simulink model "ctrl_DP"  (R2016b)
settings: Solver=ode3  StartTime=0.0  StopTime=inf  FixedStep=0.01  RelTol=1e-3  EnableMultiTasking=on
values from neighbouring files (symbols this model uses):
  C = [C1;C2;C3;C4;C5;C6]    [initfile.m]
  D = 3.0/100    (= 0.03)    [initfile.m]
  eps_c = 5    [initfile.m]
  epsilon = 0.5    [initfile.m]
  hd = c2d(H1,0.01,'foh')    [initfile.m]
  hd2 = c2d(H2,0.01,'zoh')    [initfile.m]
  I_s = 25000 /747225    (= 0.0334571246947)    [initfile.m]
  k_cc = 1    [initfile.m]
  K_omega = 0.3    [initfile.m]
  K_q1f = 0.0113    [initfile.m]
  K_q1r = K_q1f    (= 0.0113)    [initfile.m]
  K_q2f = 0.0117    [initfile.m]
  K_q2r = K_q2f    (= 0.0117)    [initfile.m]
  K_q3f = 0.0113    [initfile.m]
  K_q3r = K_q3f    (= 0.0113)    [initfile.m]
  K_q4f = 0.0169    [initfile.m]
  K_q4r = K_q4f    (= 0.0169)    [initfile.m]
  K_q5f = 0.0144    [initfile.m]
  K_q5r = K_q5f    (= 0.0144)    [initfile.m]
  K_q6f = 0.0168    [initfile.m]
  K_q6r = K_q6f    (= 0.0168)    [initfile.m]
  K_T1f = 0.3763    [initfile.m]
  K_T1r = K_T1f    (= 0.3763)    [initfile.m]
  K_T2f = 0.3901    [initfile.m]
  K_T2r = K_T2f    (= 0.3901)    [initfile.m]
  K_T3f = 0.3776    [initfile.m]
  K_T3r = K_T3f    (= 0.3776)    [initfile.m]
  K_T4f = 0.5641    [initfile.m]
  K_T4r = K_T4f    (= 0.5641)    [initfile.m]
  K_T5f = 0.4799    [initfile.m]
  K_T5r = K_T5f    (= 0.4799)    [initfile.m]
  K_T6f = 0.5588    [initfile.m]
  K_T6r = K_T6f    (= 0.5588)    [initfile.m]
  Kp = 3.3    [initfile.m]
  Max_Acceleration = 5    [initfile.m]
  Max_rotation = 12*sqrt(lambda)    [initfile.m]
  Max_thrust = 1.5    [initfile.m]
  Min_thrust = -0.8    [initfile.m]
  n_c = 5    [initfile.m]
  n_max = 152    [initfile.m]
  p_cc = 0.5    [initfile.m]
  pwm_thr1_backward = coeffvalues(ForceToPWM)    [initfile.m]
  pwm_thr1_forward = coeffvalues(ForceToPWM)    [initfile.m]
  pwm_thr2_backward = coeffvalues(ForceToPWM)    [initfile.m]
  pwm_thr2_forward = coeffvalues(ForceToPWM)    [initfile.m]
  pwm_thr3_backward = coeffvalues(ForceToPWM)    [initfile.m]
  pwm_thr3_forward = coeffvalues(ForceToPWM)    [initfile.m]
  pwm_thr4_backward = coeffvalues(ForceToPWM)    [initfile.m]
  pwm_thr4_forward = coeffvalues(ForceToPWM)    [initfile.m]
  pwm_thr5_backward = coeffvalues(ForceToPWM)    [initfile.m]
  pwm_thr5_forward = coeffvalues(ForceToPWM)    [initfile.m]
  pwm_thr6_backward = coeffvalues(ForceToPWM)    [initfile.m]
  pwm_thr6_forward = coeffvalues(ForceToPWM)    [initfile.m]
  Q_f0 = 0.3    [initfile.m]
  r_cc = 4    [initfile.m]
  Rho = Rho_m    (= 1000)    [initfile.m]
  T_pinv = T'*inv(T*T')    [initfile.m]
undefined symbols (not defined in the file or in its folder): DiscIntNeverNeededParam, Q_max, Thruster
libraries: marine_gnc x8, simulink x6, simulink_extras x3
(part 2 of 6)

== system ctrl_DP/Output ==
  u : Inport
  alpha : Inport  Port=2
  Demux : Demux  Outputs=6
  Demux1 : Demux  Outputs=6
  alpha1 : S-Function  Priority=1  FunctionName=NIVeriStandIO  Parameters=width dtype portnum stime stype btype  SFunctionDeploymentMode=off  EnableBusSupport=off  mask(NI VeriStand Outport){portnum=1, width=-1, stime=-1, dtype=auto, stype=auto, btype=0}
      mask prompts: portnum "Port number:"; width "Port dimensions (-1 for dynamically sized):"; stime "Sample time (-1 for inherited):"; dtype "Data type:"; stype "Signal type:"; btype "Block type:"
      mask help: Use this outport on any level of nested subsystems to allow NI VeriStand software to map signals to it.
      mask init:
      | NIVeriStandIO_init;
      settings: CopyFcn=NIVeriStand_MDL_functions('', 'IO_copy');  DeleteFcn=NIVeriStand_MDL_functions('', 'IO_delete');  MoveFcn=set_param(gcb, 'Mask', 'on');
      mask Callback portnum: NIVeriStand_MDL_functions('', 'IO_setportnum');
      mask TypeOptions dtype: auto | double | single | int8 | uint8 | int16 | uint16 | int32 | uint32 | boolean
      mask Callback dtype: NIVeriStand_MDL_functions('', 'IO_booleansignal');
      mask TypeOptions stype: auto | real | complex
      mask Display:
      | patch([-x x], [-y y], [.90980 .81960 .32156]);
      | plot([xrad -x x xrad], [yrad -y y yrad]);
      | fprintf('NI Out%d', portnum);
  alpha2 : S-Function  Priority=2  FunctionName=NIVeriStandIO  Parameters=width dtype portnum stime stype btype  SFunctionDeploymentMode=off  EnableBusSupport=off  mask(NI VeriStand Outport){portnum=2, width=-1, stime=-1, dtype=auto, stype=auto, btype=0}
      mask prompts: portnum "Port number:"; width "Port dimensions (-1 for dynamically sized):"; stime "Sample time (-1 for inherited):"; dtype "Data type:"; stype "Signal type:"; btype "Block type:"
      mask help: Use this outport on any level of nested subsystems to allow NI VeriStand software to map signals to it.
      mask init:
      | NIVeriStandIO_init;
      settings: CopyFcn=NIVeriStand_MDL_functions('', 'IO_copy');  DeleteFcn=NIVeriStand_MDL_functions('', 'IO_delete');  MoveFcn=set_param(gcb, 'Mask', 'on');
      mask Callback portnum: NIVeriStand_MDL_functions('', 'IO_setportnum');
      mask TypeOptions dtype: auto | double | single | int8 | uint8 | int16 | uint16 | int32 | uint32 | boolean
      mask Callback dtype: NIVeriStand_MDL_functions('', 'IO_booleansignal');
      mask TypeOptions stype: auto | real | complex
      mask Display:
      | patch([-x x], [-y y], [.90980 .81960 .32156]);
      | plot([xrad -x x xrad], [yrad -y y yrad]);
      | fprintf('NI Out%d', portnum);
  alpha3 : S-Function  Priority=3  FunctionName=NIVeriStandIO  Parameters=width dtype portnum stime stype btype  SFunctionDeploymentMode=off  EnableBusSupport=off  mask(NI VeriStand Outport){portnum=3, width=-1, stime=-1, dtype=auto, stype=auto, btype=0}
      mask prompts: portnum "Port number:"; width "Port dimensions (-1 for dynamically sized):"; stime "Sample time (-1 for inherited):"; dtype "Data type:"; stype "Signal type:"; btype "Block type:"
      mask help: Use this outport on any level of nested subsystems to allow NI VeriStand software to map signals to it.
      mask init:
      | NIVeriStandIO_init;
      settings: CopyFcn=NIVeriStand_MDL_functions('', 'IO_copy');  DeleteFcn=NIVeriStand_MDL_functions('', 'IO_delete');  MoveFcn=set_param(gcb, 'Mask', 'on');
      mask Callback portnum: NIVeriStand_MDL_functions('', 'IO_setportnum');
      mask TypeOptions dtype: auto | double | single | int8 | uint8 | int16 | uint16 | int32 | uint32 | boolean
      mask Callback dtype: NIVeriStand_MDL_functions('', 'IO_booleansignal');
      mask TypeOptions stype: auto | real | complex
      mask Display:
      | patch([-x x], [-y y], [.90980 .81960 .32156]);
      | plot([xrad -x x xrad], [yrad -y y yrad]);
      | fprintf('NI Out%d', portnum);
  alpha4 : S-Function  Priority=4  FunctionName=NIVeriStandIO  Parameters=width dtype portnum stime stype btype  SFunctionDeploymentMode=off  EnableBusSupport=off  mask(NI VeriStand Outport){portnum=4, width=-1, stime=-1, dtype=auto, stype=auto, btype=0}
      mask prompts: portnum "Port number:"; width "Port dimensions (-1 for dynamically sized):"; stime "Sample time (-1 for inherited):"; dtype "Data type:"; stype "Signal type:"; btype "Block type:"
      mask help: Use this outport on any level of nested subsystems to allow NI VeriStand software to map signals to it.
      mask init:
      | NIVeriStandIO_init;
      settings: CopyFcn=NIVeriStand_MDL_functions('', 'IO_copy');  DeleteFcn=NIVeriStand_MDL_functions('', 'IO_delete');  MoveFcn=set_param(gcb, 'Mask', 'on');
      mask Callback portnum: NIVeriStand_MDL_functions('', 'IO_setportnum');
      mask TypeOptions dtype: auto | double | single | int8 | uint8 | int16 | uint16 | int32 | uint32 | boolean
      mask Callback dtype: NIVeriStand_MDL_functions('', 'IO_booleansignal');
      mask TypeOptions stype: auto | real | complex
      mask Display:
      | patch([-x x], [-y y], [.90980 .81960 .32156]);
      | plot([xrad -x x xrad], [yrad -y y yrad]);
      | fprintf('NI Out%d', portnum);
  alpha5 : S-Function  Priority=5  FunctionName=NIVeriStandIO  Parameters=width dtype portnum stime stype btype  SFunctionDeploymentMode=off  EnableBusSupport=off  mask(NI VeriStand Outport){portnum=5, width=-1, stime=-1, dtype=auto, stype=auto, btype=0}
      mask prompts: portnum "Port number:"; width "Port dimensions (-1 for dynamically sized):"; stime "Sample time (-1 for inherited):"; dtype "Data type:"; stype "Signal type:"; btype "Block type:"
      mask help: Use this outport on any level of nested subsystems to allow NI VeriStand software to map signals to it.
      mask init:
      | NIVeriStandIO_init;
      settings: CopyFcn=NIVeriStand_MDL_functions('', 'IO_copy');  DeleteFcn=NIVeriStand_MDL_functions('', 'IO_delete');  MoveFcn=set_param(gcb, 'Mask', 'on');
      mask Callback portnum: NIVeriStand_MDL_functions('', 'IO_setportnum');
      mask TypeOptions dtype: auto | double | single | int8 | uint8 | int16 | uint16 | int32 | uint32 | boolean
      mask Callback dtype: NIVeriStand_MDL_functions('', 'IO_booleansignal');
      mask TypeOptions stype: auto | real | complex
      mask Display:
      | patch([-x x], [-y y], [.90980 .81960 .32156]);
      | plot([xrad -x x xrad], [yrad -y y yrad]);
      | fprintf('NI Out%d', portnum);
  alpha6 : S-Function  Priority=6  FunctionName=NIVeriStandIO  Parameters=width dtype portnum stime stype btype  SFunctionDeploymentMode=off  EnableBusSupport=off  mask(NI VeriStand Outport){portnum=6, width=-1, stime=-1, dtype=auto, stype=auto, btype=0}
      mask prompts: portnum "Port number:"; width "Port dimensions (-1 for dynamically sized):"; stime "Sample time (-1 for inherited):"; dtype "Data type:"; stype "Signal type:"; btype "Block type:"
      mask help: Use this outport on any level of nested subsystems to allow NI VeriStand software to map signals to it.
      mask init:
      | NIVeriStandIO_init;
      settings: CopyFcn=NIVeriStand_MDL_functions('', 'IO_copy');  DeleteFcn=NIVeriStand_MDL_functions('', 'IO_delete');  MoveFcn=set_param(gcb, 'Mask', 'on');
      mask Callback portnum: NIVeriStand_MDL_functions('', 'IO_setportnum');
      mask TypeOptions dtype: auto | double | single | int8 | uint8 | int16 | uint16 | int32 | uint32 | boolean
      mask Callback dtype: NIVeriStand_MDL_functions('', 'IO_booleansignal');
      mask TypeOptions stype: auto | real | complex
      mask Display:
      | patch([-x x], [-y y], [.90980 .81960 .32156]);
      | plot([xrad -x x xrad], [yrad -y y yrad]);
      | fprintf('NI Out%d', portnum);
  u1 : S-Function  Priority=7  FunctionName=NIVeriStandIO  Parameters=width dtype portnum stime stype btype  SFunctionDeploymentMode=off  EnableBusSupport=off  mask(NI VeriStand Outport){portnum=7, width=-1, stime=-1, dtype=auto, stype=auto, btype=0}
      mask prompts: portnum "Port number:"; width "Port dimensions (-1 for dynamically sized):"; stime "Sample time (-1 for inherited):"; dtype "Data type:"; stype "Signal type:"; btype "Block type:"
      mask help: Use this outport on any level of nested subsystems to allow NI VeriStand software to map signals to it.
      mask init:
      | NIVeriStandIO_init;
      settings: CopyFcn=NIVeriStand_MDL_functions('', 'IO_copy');  DeleteFcn=NIVeriStand_MDL_functions('', 'IO_delete');  MoveFcn=set_param(gcb, 'Mask', 'on');
      mask Callback portnum: NIVeriStand_MDL_functions('', 'IO_setportnum');
      mask TypeOptions dtype: auto | double | single | int8 | uint8 | int16 | uint16 | int32 | uint32 | boolean
      mask Callback dtype: NIVeriStand_MDL_functions('', 'IO_booleansignal');
      mask TypeOptions stype: auto | real | complex
      mask Display:
      | patch([-x x], [-y y], [.90980 .81960 .32156]);
      | plot([xrad -x x xrad], [yrad -y y yrad]);
      | fprintf('NI Out%d', portnum);
  u2 : S-Function  Priority=8  FunctionName=NIVeriStandIO  Parameters=width dtype portnum stime stype btype  SFunctionDeploymentMode=off  EnableBusSupport=off  mask(NI VeriStand Outport){portnum=8, width=-1, stime=-1, dtype=auto, stype=auto, btype=0}
      mask prompts: portnum "Port number:"; width "Port dimensions (-1 for dynamically sized):"; stime "Sample time (-1 for inherited):"; dtype "Data type:"; stype "Signal type:"; btype "Block type:"
      mask help: Use this outport on any level of nested subsystems to allow NI VeriStand software to map signals to it.
      mask init:
      | NIVeriStandIO_init;
      settings: CopyFcn=NIVeriStand_MDL_functions('', 'IO_copy');  DeleteFcn=NIVeriStand_MDL_functions('', 'IO_delete');  MoveFcn=set_param(gcb, 'Mask', 'on');
      mask Callback portnum: NIVeriStand_MDL_functions('', 'IO_setportnum');
      mask TypeOptions dtype: auto | double | single | int8 | uint8 | int16 | uint16 | int32 | uint32 | boolean
      mask Callback dtype: NIVeriStand_MDL_functions('', 'IO_booleansignal');
      mask TypeOptions stype: auto | real | complex
      mask Display:
      | patch([-x x], [-y y], [.90980 .81960 .32156]);
      | plot([xrad -x x xrad], [yrad -y y yrad]);
      | fprintf('NI Out%d', portnum);
  u3 : S-Function  Priority=9  FunctionName=NIVeriStandIO  Parameters=width dtype portnum stime stype btype  SFunctionDeploymentMode=off  EnableBusSupport=off  mask(NI VeriStand Outport){portnum=9, width=-1, stime=-1, dtype=auto, stype=auto, btype=0}
      mask prompts: portnum "Port number:"; width "Port dimensions (-1 for dynamically sized):"; stime "Sample time (-1 for inherited):"; dtype "Data type:"; stype "Signal type:"; btype "Block type:"
      mask help: Use this outport on any level of nested subsystems to allow NI VeriStand software to map signals to it.
      mask init:
      | NIVeriStandIO_init;
      settings: CopyFcn=NIVeriStand_MDL_functions('', 'IO_copy');  DeleteFcn=NIVeriStand_MDL_functions('', 'IO_delete');  MoveFcn=set_param(gcb, 'Mask', 'on');
      mask Callback portnum: NIVeriStand_MDL_functions('', 'IO_setportnum');
      mask TypeOptions dtype: auto | double | single | int8 | uint8 | int16 | uint16 | int32 | uint32 | boolean
      mask Callback dtype: NIVeriStand_MDL_functions('', 'IO_booleansignal');
      mask TypeOptions stype: auto | real | complex
      mask Display:
      | patch([-x x], [-y y], [.90980 .81960 .32156]);
      | plot([xrad -x x xrad], [yrad -y y yrad]);
      | fprintf('NI Out%d', portnum);
  u4 : S-Function  Priority=10  FunctionName=NIVeriStandIO  Parameters=width dtype portnum stime stype btype  SFunctionDeploymentMode=off  EnableBusSupport=off  mask(NI VeriStand Outport){portnum=10, width=-1, stime=-1, dtype=auto, stype=auto, btype=0}
      mask prompts: portnum "Port number:"; width "Port dimensions (-1 for dynamically sized):"; stime "Sample time (-1 for inherited):"; dtype "Data type:"; stype "Signal type:"; btype "Block type:"
      mask help: Use this outport on any level of nested subsystems to allow NI VeriStand software to map signals to it.
      mask init:
      | NIVeriStandIO_init;
      settings: CopyFcn=NIVeriStand_MDL_functions('', 'IO_copy');  DeleteFcn=NIVeriStand_MDL_functions('', 'IO_delete');  MoveFcn=set_param(gcb, 'Mask', 'on');
      mask Callback portnum: NIVeriStand_MDL_functions('', 'IO_setportnum');
      mask TypeOptions dtype: auto | double | single | int8 | uint8 | int16 | uint16 | int32 | uint32 | boolean
      mask Callback dtype: NIVeriStand_MDL_functions('', 'IO_booleansignal');
      mask TypeOptions stype: auto | real | complex
      mask Display:
      | patch([-x x], [-y y], [.90980 .81960 .32156]);
      | plot([xrad -x x xrad], [yrad -y y yrad]);
      | fprintf('NI Out%d', portnum);
  u5 : S-Function  Priority=11  FunctionName=NIVeriStandIO  Parameters=width dtype portnum stime stype btype  SFunctionDeploymentMode=off  EnableBusSupport=off  mask(NI VeriStand Outport){portnum=11, width=-1, stime=-1, dtype=auto, stype=auto, btype=0}
      mask prompts: portnum "Port number:"; width "Port dimensions (-1 for dynamically sized):"; stime "Sample time (-1 for inherited):"; dtype "Data type:"; stype "Signal type:"; btype "Block type:"
      mask help: Use this outport on any level of nested subsystems to allow NI VeriStand software to map signals to it.
      mask init:
      | NIVeriStandIO_init;
      settings: CopyFcn=NIVeriStand_MDL_functions('', 'IO_copy');  DeleteFcn=NIVeriStand_MDL_functions('', 'IO_delete');  MoveFcn=set_param(gcb, 'Mask', 'on');
      mask Callback portnum: NIVeriStand_MDL_functions('', 'IO_setportnum');
      mask TypeOptions dtype: auto | double | single | int8 | uint8 | int16 | uint16 | int32 | uint32 | boolean
      mask Callback dtype: NIVeriStand_MDL_functions('', 'IO_booleansignal');
      mask TypeOptions stype: auto | real | complex
      mask Display:
      | patch([-x x], [-y y], [.90980 .81960 .32156]);
      | plot([xrad -x x xrad], [yrad -y y yrad]);
      | fprintf('NI Out%d', portnum);
  u6 : S-Function  Priority=12  FunctionName=NIVeriStandIO  Parameters=width dtype portnum stime stype btype  SFunctionDeploymentMode=off  EnableBusSupport=off  mask(NI VeriStand Outport){portnum=12, width=-1, stime=-1, dtype=auto, stype=auto, btype=0}
      mask prompts: portnum "Port number:"; width "Port dimensions (-1 for dynamically sized):"; stime "Sample time (-1 for inherited):"; dtype "Data type:"; stype "Signal type:"; btype "Block type:"
      mask help: Use this outport on any level of nested subsystems to allow NI VeriStand software to map signals to it.
      mask init:
      | NIVeriStandIO_init;
      settings: CopyFcn=NIVeriStand_MDL_functions('', 'IO_copy');  DeleteFcn=NIVeriStand_MDL_functions('', 'IO_delete');  MoveFcn=set_param(gcb, 'Mask', 'on');
      mask Callback portnum: NIVeriStand_MDL_functions('', 'IO_setportnum');
      mask TypeOptions dtype: auto | double | single | int8 | uint8 | int16 | uint16 | int32 | uint32 | boolean
      mask Callback dtype: NIVeriStand_MDL_functions('', 'IO_booleansignal');
      mask TypeOptions stype: auto | real | complex
      mask Display:
      | patch([-x x], [-y y], [.90980 .81960 .32156]);
      | plot([xrad -x x xrad], [yrad -y y yrad]);
      | fprintf('NI Out%d', portnum);
  wires:
  u/1 -> Demux/1
  Demux/1 -> u1/1
  Demux/2 -> u2/1
  Demux/3 -> u3/1
  Demux/4 -> u4/1
  Demux/5 -> u5/1
  Demux/6 -> u6/1
  alpha/1 -> Demux1/1
  Demux1/1 -> alpha1/1
  Demux1/2 -> alpha2/1
  Demux1/3 -> alpha3/1
  Demux1/4 -> alpha4/1
  Demux1/5 -> alpha5/1
  Demux1/6 -> alpha6/1

== system ctrl_DP/Projection [-pi,pi] to [-inf,inf] + shortest rotation ==
  alpha_pipi : Inport
  MATLAB Function11 : MATLAB Function  TreatAsAtomicUnit=on
  Memory4 : Memory  X0=[0 0 0 0 0 0]'
  alpha_infinf : Outport
  wires:
  alpha_pipi/1 -> MATLAB Function11/2(alpha_pipi)
  MATLAB Function11/1(alpha_infinf) -> Memory4/1, alpha_infinf/1
  Memory4/1 -> MATLAB Function11/1(alpha_prev)

== system ctrl_DP/Thrust allocation ==
  tau : Inport
  Angles : Inport  Port=2
  "  Thrust calculated" : Selector  InputPortWidth=12  IndexOptions=Index vector (dialog)  Indices=[7 8 9 10 11 12]  OutputSizes=1
  " Angle calculated" : Selector  InputPortWidth=12  IndexOptions=Index vector (dialog)  Indices=[1 2 3 4 5 6]  OutputSizes=1
  Angle_controller : S-Function  Priority=2  FunctionName=NIVeriStandIO  Parameters=width dtype portnum stime stype btype  SFunctionDeploymentMode=off  EnableBusSupport=off  mask(NI VeriStand Inport){portnum=2, width=-1, stime=-1, dtype=auto, stype=auto, btype=1}
      mask prompts: portnum "Port number:"; width "Port dimensions (-1 for dynamically sized):"; stime "Sample time (-1 for inherited):"; dtype "Data type:"; stype "Signal type:"; btype "Block type:"
      mask help: Use this inport on any level of nested subsystems to allow NI VeriStand software to map signals to it.
      mask init:
      | NIVeriStandIO_init;
      settings: CopyFcn=NIVeriStand_MDL_functions('', 'IO_copy');  DeleteFcn=NIVeriStand_MDL_functions('', 'IO_delete');  MoveFcn=set_param(gcb, 'Mask', 'on');
      mask Callback portnum: NIVeriStand_MDL_functions('', 'IO_setportnum');
      mask TypeOptions dtype: auto | double | single | int8 | uint8 | int16 | uint16 | int32 | uint32 | boolean
      mask Callback dtype: NIVeriStand_MDL_functions('', 'IO_booleansignal');
      mask TypeOptions stype: auto | real | complex
      mask Display:
      | patch([-x x], [-y y], [.90980 .81960 .32156]);
      | plot([xrad -x x xrad], [yrad -y y yrad]);
      | fprintf('NI In%d', portnum);
  C : Constant  Value=C
  Choosing Fixed / Azimuth angle : Switch  Threshold=1
  Constant to avoid singularities : Constant  Value=eps
  MATLAB Function : MATLAB Function  TreatAsAtomicUnit=on
  Mux : Mux  Inputs=3
  Mux2 : Mux  Inputs=2
  Optimal angle path and constraints on rotation speed : Subsystem  TreatAsAtomicUnit=on
  Radians to Degrees : simulink_extras/Transformations/Radians to Degrees
  X-position Thruster : Constant  Value=[Thruster.T1(1) Thruster.T2(1) Thruster.T3(1) Thruster.T4(1) Thruster.T5(1) Thruster.T6(1)]
  Y-position Thruster : Constant  Value=[Thruster.T1(2) Thruster.T2(2) Thruster.T3(2) Thruster.T4(2) Thruster.T5(2) Thruster.T6(2)]
  angle between [-180 180] : MATLAB Function  TreatAsAtomicUnit=on
  constant angle : Constant  Value=[Thruster.T1(3) Thruster.T2(3) Thruster.T3(3) Thruster.T4(3) Thruster.T5(3) Thruster.T6(3)]
  reset : S-Function  Priority=1  FunctionName=NIVeriStandIO  Parameters=width dtype portnum stime stype btype  SFunctionDeploymentMode=off  EnableBusSupport=off  mask(NI VeriStand Inport){portnum=1, width=-1, stime=-1, dtype=auto, stype=auto, btype=1}
      mask prompts: portnum "Port number:"; width "Port dimensions (-1 for dynamically sized):"; stime "Sample time (-1 for inherited):"; dtype "Data type:"; stype "Signal type:"; btype "Block type:"
      mask help: Use this inport on any level of nested subsystems to allow NI VeriStand software to map signals to it.
      mask init:
      | NIVeriStandIO_init;
      settings: CopyFcn=NIVeriStand_MDL_functions('', 'IO_copy');  DeleteFcn=NIVeriStand_MDL_functions('', 'IO_delete');  MoveFcn=set_param(gcb, 'Mask', 'on');
      mask Callback portnum: NIVeriStand_MDL_functions('', 'IO_setportnum');
      mask TypeOptions dtype: auto | double | single | int8 | uint8 | int16 | uint16 | int32 | uint32 | boolean
      mask Callback dtype: NIVeriStand_MDL_functions('', 'IO_booleansignal');
      mask TypeOptions stype: auto | real | complex
      mask Display:
      | patch([-x x], [-y y], [.90980 .81960 .32156]);
      | plot([xrad -x x xrad], [yrad -y y yrad]);
      | fprintf('NI In%d', portnum);
  u_d & angle : Outport
  wires:
  Angle_controller/1 -> Choosing Fixed / Azimuth angle/2
  Constant to avoid singularities/1 -> Mux/3
  " Angle calculated"/1 -> Choosing Fixed / Azimuth angle/1
  Mux2/1 -> u_d & angle/1
  "  Thrust calculated"/1 -> Mux2/2
  tau/1 -> Mux/1
  Choosing Fixed / Azimuth angle/1 -> Optimal angle path and constraints on rotation speed/1(Desired Angle)
  Angles/1 -> angle between [-180 180]/1(angle)
  Optimal angle path and constraints on rotation speed/1(commanded Angle) -> Mux2/1
  constant angle/1 -> Optimal angle path and constraints on rotation speed/2("initial angle "), Choosing Fixed / Azimuth angle/3
  Radians to Degrees/1 -> Mux/2
  reset/1 -> Optimal angle path and constraints on rotation speed/3(reset)
  X-position Thruster/1 -> MATLAB Function/2(ThrusterPosX)
  Y-position Thruster/1 -> MATLAB Function/3(ThrusterPosY)
  C/1 -> MATLAB Function/4(C)
  MATLAB Function/1(sys) -> " Angle calculated"/1, "  Thrust calculated"/1
  Mux/1 -> MATLAB Function/1(u)
  angle between [-180 180]/1(y) -> Radians to Degrees/1

== system ctrl_DP/Thrust allocation: Pseudo-inverse of extended thrust configuration matrix ==
  tau [N] : Inport
  Gain : Gain  Gain=T_pinv  Multiplication=Matrix(K*u)
  MATLAB Function11 : MATLAB Function  TreatAsAtomicUnit=on
  u [N] : Outport
  alpha [rad] : Outport  Port=2
  wires:
  MATLAB Function11/2(alpha) -> alpha [rad]/1
  tau [N]/1 -> Gain/1
  Gain/1 -> MATLAB Function11/1(u_e)  "u_e"
  MATLAB Function11/1(u) -> u [N]/1

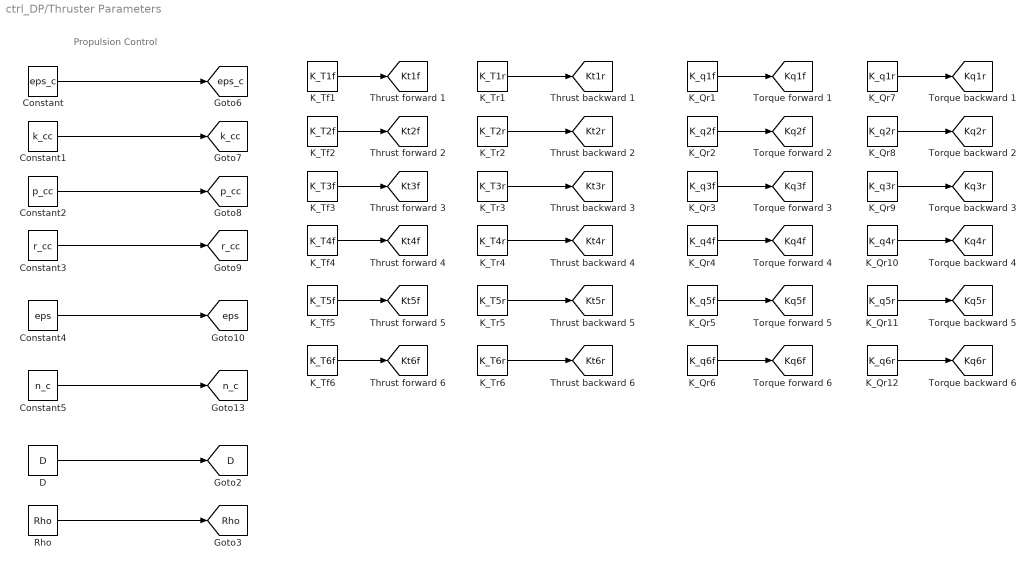
== system ctrl_DP/Thruster Parameters  ==
  note: Propulsion Control
  Constant : Constant  Value=eps_c
  Constant1 : Constant  Value=k_cc
  Constant2 : Constant  Value=p_cc
  Constant3 : Constant  Value=r_cc
  Constant4 : Constant  Value=eps
  Constant5 : Constant  Value=n_c
  D : Constant  Value=D
  K_Qr1 : Constant  Value=K_q1f
  K_Qr10 : Constant  Value=K_q4r
  K_Qr11 : Constant  Value=K_q5r
  K_Qr12 : Constant  Value=K_q6r
  K_Qr2 : Constant  Value=K_q2f
  K_Qr3 : Constant  Value=K_q3f
  K_Qr4 : Constant  Value=K_q4f
  K_Qr5 : Constant  Value=K_q5f
  K_Qr6 : Constant  Value=K_q6f
  K_Qr7 : Constant  Value=K_q1r
  K_Qr8 : Constant  Value=K_q2r
  K_Qr9 : Constant  Value=K_q3r
  K_Tf1 : Constant  Value=K_T1f
  K_Tf2 : Constant  Value=K_T2f
  K_Tf3 : Constant  Value=K_T3f
  K_Tf4 : Constant  Value=K_T4f
  K_Tf5 : Constant  Value=K_T5f
  K_Tf6 : Constant  Value=K_T6f
  K_Tr1 : Constant  Value=K_T1r
  K_Tr2 : Constant  Value=K_T2r
  K_Tr3 : Constant  Value=K_T3r
  K_Tr4 : Constant  Value=K_T4r
  K_Tr5 : Constant  Value=K_T5r
  K_Tr6 : Constant  Value=K_T6r
  Rho : Constant  Value=Rho
  tag scope: D=global, Kq1f=global, Kq1r=global, Kq2f=global, Kq2r=global, Kq3f=global, Kq3r=global, Kq4f=global, Kq4r=global, Kq5f=global, Kq5r=global, Kq6f=global, Kq6r=global, Kt1f=global, Kt1r=global, Kt2f=global, Kt2r=global, Kt3f=global, Kt3r=global, Kt4f=global, Kt4r=global, Kt5f=global, Kt5r=global, Kt6f=global, Kt6r=global, Rho=global, eps=global, eps_c=global, k_cc=global, n_c=global, p_cc=global, r_cc=global
  wires:
  D/1 -> [D]
  Rho/1 -> [Rho]
  Constant/1 -> [eps_c]
  Constant1/1 -> [k_cc]
  Constant2/1 -> [p_cc]
  Constant3/1 -> [r_cc]
  Constant4/1 -> [eps]
  Constant5/1 -> [n_c]
  K_Tf1/1 -> [Kt1f]
  K_Tf6/1 -> [Kt6f]
  K_Tf5/1 -> [Kt5f]
  K_Tf4/1 -> [Kt4f]
  K_Tf3/1 -> [Kt3f]
  K_Tf2/1 -> [Kt2f]
  K_Tr1/1 -> [Kt1r]
  K_Tr6/1 -> [Kt6r]
  K_Tr5/1 -> [Kt5r]
  K_Tr4/1 -> [Kt4r]
  K_Tr2/1 -> [Kt2r]
  K_Tr3/1 -> [Kt3r]
  K_Qr1/1 -> [Kq1f]
  K_Qr2/1 -> [Kq2f]
  K_Qr3/1 -> [Kq3f]
  K_Qr4/1 -> [Kq4f]
  K_Qr5/1 -> [Kq5f]
  K_Qr6/1 -> [Kq6f]
  K_Qr7/1 -> [Kq1r]
  K_Qr8/1 -> [Kq2r]
  K_Qr9/1 -> [Kq3r]
  K_Qr10/1 -> [Kq4r]
  K_Qr11/1 -> [Kq5r]
  K_Qr12/1 -> [Kq6r]

== system ctrl_DP/Thruster control  ==
  "Desired thrust and angle " : Inport
  Delay : Delay  DelayLength=1  InitialCondition=0
  Demux : Demux  Outputs=12
  Mapping shaft speed and thrust : Selector  InputPortWidth=12  IndexOptions=Index vector (dialog)  Indices="[1 7 2  8 3 9 4 10 5 11 6 12]"  OutputSizes=1
  Mux : Mux  Inputs=12
  Mux1 : Mux  Inputs=2
  Selecting Desired thrust1 : Selector  InputPortWidth=12  IndexOptions=Index vector (dialog)  Indices=[7 8 9 10 11 12]  OutputSizes=1
  Selecting actual angle : Selector  InputPortWidth=12  IndexOptions=Index vector (dialog)  Indices=[1 2 3 4 5 6]  OutputSizes=1
  Subsystem1 : Subsystem
  Thrust and Shaft speed mapped to PWM : Subsystem
  Thruster 1 : Subsystem
      settings: AttributesFormatString=%<MinAlgLoopOccurrences>
  Thruster 2 : Subsystem
      settings: AttributesFormatString=%<MinAlgLoopOccurrences>
  Thruster 3 : Subsystem
      settings: AttributesFormatString=%<MinAlgLoopOccurrences>
  Thruster 4 : Subsystem
      settings: AttributesFormatString=%<MinAlgLoopOccurrences>
  Thruster 5 : Subsystem
      settings: AttributesFormatString=%<MinAlgLoopOccurrences>
  Thruster 6 : Subsystem
      settings: AttributesFormatString=%<MinAlgLoopOccurrences>
  "Commanded pwm " : Outport
  Commanded angle : Outport  Port=2
  Commanded thrust : Outport  Port=3
  wires:
  Selecting actual angle/1 -> Subsystem1/1(Calculated angles)
  "Desired thrust and angle "/1 -> Selecting actual angle/1, Selecting Desired thrust1/1
  Subsystem1/1(Commanded angles) -> Commanded angle/1
  Thrust and Shaft speed mapped to PWM/1(pwm) -> "Commanded pwm "/1
  Thrust and Shaft speed mapped to PWM/2(Force) -> Commanded thrust/1
  Thrust and Shaft speed mapped to PWM/3("Shaft speed ") -> Delay/1
  Thruster 1/1("Commanded thrust ") -> Mux/1
  Mux/1 -> Thrust and Shaft speed mapped to PWM/1(Calculated thrust)
  Mux1/1 -> Mapping shaft speed and thrust/1
  Delay/1 -> Mux1/2
  Mapping shaft speed and thrust/1 -> Demux/1
  Thruster 1/2(Shaft speed) -> Mux/2
  Demux/2 -> Thruster 1/2(shaft speed)
  Demux/1 -> Thruster 1/1(Desired thrust 1)
  Thruster 2/1("Commanded thrust ") -> Mux/3
  Demux/3 -> Thruster 2/1(Desired thrust 1)
  Demux/4 -> Thruster 2/2(shaft speed)
  Demux/5 -> Thruster 3/1(Desired thrust 1)
  Demux/6 -> Thruster 3/2(shaft speed)
  Demux/7 -> Thruster 4/1(Desired thrust 1)
  Demux/8 -> Thruster 4/2(shaft speed)
  Demux/9 -> Thruster 5/1(Desired thrust 1)
  Demux/10 -> Thruster 5/2(shaft speed)
  Demux/11 -> Thruster 6/1(Desired thrust 1)
  Demux/12 -> Thruster 6/2(shaft speed)
  Thruster 2/2(Shaft speed) -> Mux/4
  Thruster 3/1("Commanded thrust ") -> Mux/5
  Thruster 3/2(Shaft speed) -> Mux/6
  Thruster 4/1("Commanded thrust ") -> Mux/7
  Thruster 4/2(Shaft speed) -> Mux/8
  Thruster 5/1("Commanded thrust ") -> Mux/9
  Thruster 5/2(Shaft speed) -> Mux/10
  Thruster 6/1("Commanded thrust ") -> Mux/11
  Thruster 6/2(Shaft speed) -> Mux/12
  Selecting Desired thrust1/1 -> Mux1/1

== system ctrl_DP/Thruster measurment ==
  Mux1 : Mux  Inputs=6
  thr_angle_1 : S-Function  Priority=1  FunctionName=NIVeriStandIO  Parameters=width dtype portnum stime stype btype  SFunctionDeploymentMode=off  EnableBusSupport=off  mask(NI VeriStand Inport){portnum=1, width=-1, stime=-1, dtype=auto, stype=auto, btype=1}
      mask prompts: portnum "Port number:"; width "Port dimensions (-1 for dynamically sized):"; stime "Sample time (-1 for inherited):"; dtype "Data type:"; stype "Signal type:"; btype "Block type:"
      mask help: Use this inport on any level of nested subsystems to allow NI VeriStand software to map signals to it.
      mask init:
      | NIVeriStandIO_init;
      settings: CopyFcn=NIVeriStand_MDL_functions('', 'IO_copy');  DeleteFcn=NIVeriStand_MDL_functions('', 'IO_delete');  MoveFcn=set_param(gcb, 'Mask', 'on');
      mask Callback portnum: NIVeriStand_MDL_functions('', 'IO_setportnum');
      mask TypeOptions dtype: auto | double | single | int8 | uint8 | int16 | uint16 | int32 | uint32 | boolean
      mask Callback dtype: NIVeriStand_MDL_functions('', 'IO_booleansignal');
      mask TypeOptions stype: auto | real | complex
      mask Display:
      | patch([-x x], [-y y], [.90980 .81960 .32156]);
      | plot([xrad -x x xrad], [yrad -y y yrad]);
      | fprintf('NI In%d', portnum);
  thr_angle_2 : S-Function  Priority=2  FunctionName=NIVeriStandIO  Parameters=width dtype portnum stime stype btype  SFunctionDeploymentMode=off  EnableBusSupport=off  mask(NI VeriStand Inport){portnum=2, width=-1, stime=-1, dtype=auto, stype=auto, btype=1}
      mask prompts: portnum "Port number:"; width "Port dimensions (-1 for dynamically sized):"; stime "Sample time (-1 for inherited):"; dtype "Data type:"; stype "Signal type:"; btype "Block type:"
      mask help: Use this inport on any level of nested subsystems to allow NI VeriStand software to map signals to it.
      mask init:
      | NIVeriStandIO_init;
      settings: CopyFcn=NIVeriStand_MDL_functions('', 'IO_copy');  DeleteFcn=NIVeriStand_MDL_functions('', 'IO_delete');  MoveFcn=set_param(gcb, 'Mask', 'on');
      mask Callback portnum: NIVeriStand_MDL_functions('', 'IO_setportnum');
      mask TypeOptions dtype: auto | double | single | int8 | uint8 | int16 | uint16 | int32 | uint32 | boolean
      mask Callback dtype: NIVeriStand_MDL_functions('', 'IO_booleansignal');
      mask TypeOptions stype: auto | real | complex
      mask Display:
      | patch([-x x], [-y y], [.90980 .81960 .32156]);
      | plot([xrad -x x xrad], [yrad -y y yrad]);
      | fprintf('NI In%d', portnum);
  thr_angle_3 : S-Function  Priority=3  FunctionName=NIVeriStandIO  Parameters=width dtype portnum stime stype btype  SFunctionDeploymentMode=off  EnableBusSupport=off  mask(NI VeriStand Inport){portnum=3, width=-1, stime=-1, dtype=auto, stype=auto, btype=1}
      mask prompts: portnum "Port number:"; width "Port dimensions (-1 for dynamically sized):"; stime "Sample time (-1 for inherited):"; dtype "Data type:"; stype "Signal type:"; btype "Block type:"
      mask help: Use this inport on any level of nested subsystems to allow NI VeriStand software to map signals to it.
      mask init:
      | NIVeriStandIO_init;
      settings: CopyFcn=NIVeriStand_MDL_functions('', 'IO_copy');  DeleteFcn=NIVeriStand_MDL_functions('', 'IO_delete');  MoveFcn=set_param(gcb, 'Mask', 'on');
      mask Callback portnum: NIVeriStand_MDL_functions('', 'IO_setportnum');
      mask TypeOptions dtype: auto | double | single | int8 | uint8 | int16 | uint16 | int32 | uint32 | boolean
      mask Callback dtype: NIVeriStand_MDL_functions('', 'IO_booleansignal');
      mask TypeOptions stype: auto | real | complex
      mask Display:
      | patch([-x x], [-y y], [.90980 .81960 .32156]);
      | plot([xrad -x x xrad], [yrad -y y yrad]);
      | fprintf('NI In%d', portnum);
  thr_angle_4 : S-Function  Priority=4  FunctionName=NIVeriStandIO  Parameters=width dtype portnum stime stype btype  SFunctionDeploymentMode=off  EnableBusSupport=off  mask(NI VeriStand Inport){portnum=4, width=-1, stime=-1, dtype=auto, stype=auto, btype=1}
      mask prompts: portnum "Port number:"; width "Port dimensions (-1 for dynamically sized):"; stime "Sample time (-1 for inherited):"; dtype "Data type:"; stype "Signal type:"; btype "Block type:"
      mask help: Use this inport on any level of nested subsystems to allow NI VeriStand software to map signals to it.
      mask init:
      | NIVeriStandIO_init;
      settings: CopyFcn=NIVeriStand_MDL_functions('', 'IO_copy');  DeleteFcn=NIVeriStand_MDL_functions('', 'IO_delete');  MoveFcn=set_param(gcb, 'Mask', 'on');
      mask Callback portnum: NIVeriStand_MDL_functions('', 'IO_setportnum');
      mask TypeOptions dtype: auto | double | single | int8 | uint8 | int16 | uint16 | int32 | uint32 | boolean
      mask Callback dtype: NIVeriStand_MDL_functions('', 'IO_booleansignal');
      mask TypeOptions stype: auto | real | complex
      mask Display:
      | patch([-x x], [-y y], [.90980 .81960 .32156]);
      | plot([xrad -x x xrad], [yrad -y y yrad]);
      | fprintf('NI In%d', portnum);
  thr_angle_5 : S-Function  Priority=5  FunctionName=NIVeriStandIO  Parameters=width dtype portnum stime stype btype  SFunctionDeploymentMode=off  EnableBusSupport=off  mask(NI VeriStand Inport){portnum=5, width=-1, stime=-1, dtype=auto, stype=auto, btype=1}
      mask prompts: portnum "Port number:"; width "Port dimensions (-1 for dynamically sized):"; stime "Sample time (-1 for inherited):"; dtype "Data type:"; stype "Signal type:"; btype "Block type:"
      mask help: Use this inport on any level of nested subsystems to allow NI VeriStand software to map signals to it.
      mask init:
      | NIVeriStandIO_init;
      settings: CopyFcn=NIVeriStand_MDL_functions('', 'IO_copy');  DeleteFcn=NIVeriStand_MDL_functions('', 'IO_delete');  MoveFcn=set_param(gcb, 'Mask', 'on');
      mask Callback portnum: NIVeriStand_MDL_functions('', 'IO_setportnum');
      mask TypeOptions dtype: auto | double | single | int8 | uint8 | int16 | uint16 | int32 | uint32 | boolean
      mask Callback dtype: NIVeriStand_MDL_functions('', 'IO_booleansignal');
      mask TypeOptions stype: auto | real | complex
      mask Display:
      | patch([-x x], [-y y], [.90980 .81960 .32156]);
      | plot([xrad -x x xrad], [yrad -y y yrad]);
      | fprintf('NI In%d', portnum);
  thr_angle_6 : S-Function  Priority=6  FunctionName=NIVeriStandIO  Parameters=width dtype portnum stime stype btype  SFunctionDeploymentMode=off  EnableBusSupport=off  mask(NI VeriStand Inport){portnum=6, width=-1, stime=-1, dtype=auto, stype=auto, btype=1}
      mask prompts: portnum "Port number:"; width "Port dimensions (-1 for dynamically sized):"; stime "Sample time (-1 for inherited):"; dtype "Data type:"; stype "Signal type:"; btype "Block type:"
      mask help: Use this inport on any level of nested subsystems to allow NI VeriStand software to map signals to it.
      mask init:
      | NIVeriStandIO_init;
      settings: CopyFcn=NIVeriStand_MDL_functions('', 'IO_copy');  DeleteFcn=NIVeriStand_MDL_functions('', 'IO_delete');  MoveFcn=set_param(gcb, 'Mask', 'on');
      mask Callback portnum: NIVeriStand_MDL_functions('', 'IO_setportnum');
      mask TypeOptions dtype: auto | double | single | int8 | uint8 | int16 | uint16 | int32 | uint32 | boolean
      mask Callback dtype: NIVeriStand_MDL_functions('', 'IO_booleansignal');
      mask TypeOptions stype: auto | real | complex
      mask Display:
      | patch([-x x], [-y y], [.90980 .81960 .32156]);
      | plot([xrad -x x xrad], [yrad -y y yrad]);
      | fprintf('NI In%d', portnum);
  alpha_m : Outport
  wires:
  thr_angle_3/1 -> Mux1/3
  thr_angle_1/1 -> Mux1/1
  Mux1/1 -> alpha_m/1
  thr_angle_5/1 -> Mux1/5
  thr_angle_4/1 -> Mux1/4
  thr_angle_6/1 -> Mux1/6
  thr_angle_2/1 -> Mux1/2

== system ctrl_DP/eta_QTM ==
  note: Measurements in mm and degrees
  note: x
  note: r
  Constant1 : Constant  Value=2*pi
  Gain1 : Gain  Gain=1/1000
  Gain6 : Gain  Gain=pi  SaturateOnIntegerOverflow=on  OutDataTypeStr=Inherit: Same as input  ParamDataTypeStr=Inherit: Same as input
  Math Function : Math  Operator=rem  SaturateOnIntegerOverflow=on
  Saturation : Saturate  UpperLimit=1e10  LowerLimit=-1e10
  Sign : Signum
  Sum : Sum  Inputs=|+-  SaturateOnIntegerOverflow=on
  Sum1 : Sum  Inputs=|++  SaturateOnIntegerOverflow=on
  deg2rad : Gain  Gain=pi/180
  mm2m : Gain  Gain=1/1000
  psi_m : S-Function  Priority=3  FunctionName=NIVeriStandIO  Parameters=width dtype portnum stime stype btype  SFunctionDeploymentMode=off  EnableBusSupport=off  mask(NI VeriStand Inport){portnum=3, width=-1, stime=-1, dtype=auto, stype=auto, btype=1}
      mask prompts: portnum "Port number:"; width "Port dimensions (-1 for dynamically sized):"; stime "Sample time (-1 for inherited):"; dtype "Data type:"; stype "Signal type:"; btype "Block type:"
      mask help: Use this inport on any level of nested subsystems to allow NI VeriStand software to map signals to it.
      mask init:
      | NIVeriStandIO_init;
      settings: CopyFcn=NIVeriStand_MDL_functions('', 'IO_copy');  DeleteFcn=NIVeriStand_MDL_functions('', 'IO_delete');  MoveFcn=set_param(gcb, 'Mask', 'on');
      mask Callback portnum: NIVeriStand_MDL_functions('', 'IO_setportnum');
      mask TypeOptions dtype: auto | double | single | int8 | uint8 | int16 | uint16 | int32 | uint32 | boolean
      mask Callback dtype: NIVeriStand_MDL_functions('', 'IO_booleansignal');
      mask TypeOptions stype: auto | real | complex
      mask Display:
      | patch([-x x], [-y y], [.90980 .81960 .32156]);
      | plot([xrad -x x xrad], [yrad -y y yrad]);
      | fprintf('NI In%d', portnum);
  x_m : S-Function  Priority=1  FunctionName=NIVeriStandIO  Parameters=width dtype portnum stime stype btype  SFunctionDeploymentMode=off  EnableBusSupport=off  mask(NI VeriStand Inport){portnum=1, width=-1, stime=-1, dtype=auto, stype=auto, btype=1}
      mask prompts: portnum "Port number:"; width "Port dimensions (-1 for dynamically sized):"; stime "Sample time (-1 for inherited):"; dtype "Data type:"; stype "Signal type:"; btype "Block type:"
      mask help: Use this inport on any level of nested subsystems to allow NI VeriStand software to map signals to it.
      mask init:
      | NIVeriStandIO_init;
      settings: CopyFcn=NIVeriStand_MDL_functions('', 'IO_copy');  DeleteFcn=NIVeriStand_MDL_functions('', 'IO_delete');  MoveFcn=set_param(gcb, 'Mask', 'on');
      mask Callback portnum: NIVeriStand_MDL_functions('', 'IO_setportnum');
      mask TypeOptions dtype: auto | double | single | int8 | uint8 | int16 | uint16 | int32 | uint32 | boolean
      mask Callback dtype: NIVeriStand_MDL_functions('', 'IO_booleansignal');
      mask TypeOptions stype: auto | real | complex
      mask Display:
      | patch([-x x], [-y y], [.90980 .81960 .32156]);
      | plot([xrad -x x xrad], [yrad -y y yrad]);
      | fprintf('NI In%d', portnum);
  y_m : S-Function  Priority=2  FunctionName=NIVeriStandIO  Parameters=width dtype portnum stime stype btype  SFunctionDeploymentMode=off  EnableBusSupport=off  mask(NI VeriStand Inport){portnum=2, width=-1, stime=-1, dtype=auto, stype=auto, btype=1}
      mask prompts: portnum "Port number:"; width "Port dimensions (-1 for dynamically sized):"; stime "Sample time (-1 for inherited):"; dtype "Data type:"; stype "Signal type:"; btype "Block type:"
      mask help: Use this inport on any level of nested subsystems to allow NI VeriStand software to map signals to it.
      mask init:
      | NIVeriStandIO_init;
      settings: CopyFcn=NIVeriStand_MDL_functions('', 'IO_copy');  DeleteFcn=NIVeriStand_MDL_functions('', 'IO_delete');  MoveFcn=set_param(gcb, 'Mask', 'on');
      mask Callback portnum: NIVeriStand_MDL_functions('', 'IO_setportnum');
      mask TypeOptions dtype: auto | double | single | int8 | uint8 | int16 | uint16 | int32 | uint32 | boolean
      mask Callback dtype: NIVeriStand_MDL_functions('', 'IO_booleansignal');
      mask TypeOptions stype: auto | real | complex
      mask Display:
      | patch([-x x], [-y y], [.90980 .81960 .32156]);
      | plot([xrad -x x xrad], [yrad -y y yrad]);
      | fprintf('NI In%d', portnum);
  x_QTM [m] : Outport
  y_QTM [m] : Outport  Port=2
  psi_QTM [rad] : Outport  Port=3
  wires:
  y_m/1 -> Gain1/1
  x_m/1 -> mm2m/1
  mm2m/1 -> x_QTM [m]/1
  Gain1/1 -> y_QTM [m]/1
  deg2rad/1 -> Saturation/1
  Math Function/1 -> Sum/1
  Saturation/1 -> Sum1/1, Sign/1
  Sum/1 -> psi_QTM [rad]/1
  Gain6/1 -> Sum/2, Sum1/2
  Constant1/1 -> Math Function/2
  Sum1/1 -> Math Function/1
  Sign/1 -> Gain6/1
  psi_m/1 -> deg2rad/1  "[-180,180] [deg]"

== system ctrl_DP/Control/eta_tilde ==
  eta_tilde : Inport
  Demux : Demux  Outputs=3
  psi_tilde : S-Function  Priority=3  FunctionName=NIVeriStandIO  Parameters=width dtype portnum stime stype btype  SFunctionDeploymentMode=off  EnableBusSupport=off  mask(NI VeriStand Outport){portnum=3, width=-1, stime=-1, dtype=auto, stype=auto, btype=0}
      mask prompts: portnum "Port number:"; width "Port dimensions (-1 for dynamically sized):"; stime "Sample time (-1 for inherited):"; dtype "Data type:"; stype "Signal type:"; btype "Block type:"
      mask help: Use this outport on any level of nested subsystems to allow NI VeriStand software to map signals to it.
      mask init:
      | NIVeriStandIO_init;
      settings: CopyFcn=NIVeriStand_MDL_functions('', 'IO_copy');  DeleteFcn=NIVeriStand_MDL_functions('', 'IO_delete');  MoveFcn=set_param(gcb, 'Mask', 'on');
      mask Callback portnum: NIVeriStand_MDL_functions('', 'IO_setportnum');
      mask TypeOptions dtype: auto | double | single | int8 | uint8 | int16 | uint16 | int32 | uint32 | boolean
      mask Callback dtype: NIVeriStand_MDL_functions('', 'IO_booleansignal');
      mask TypeOptions stype: auto | real | complex
      mask Display:
      | patch([-x x], [-y y], [.90980 .81960 .32156]);
      | plot([xrad -x x xrad], [yrad -y y yrad]);
      | fprintf('NI Out%d', portnum);
  x_tilde : S-Function  Priority=1  FunctionName=NIVeriStandIO  Parameters=width dtype portnum stime stype btype  SFunctionDeploymentMode=off  EnableBusSupport=off  mask(NI VeriStand Outport){portnum=1, width=-1, stime=-1, dtype=auto, stype=auto, btype=0}
      mask prompts: portnum "Port number:"; width "Port dimensions (-1 for dynamically sized):"; stime "Sample time (-1 for inherited):"; dtype "Data type:"; stype "Signal type:"; btype "Block type:"
      mask help: Use this outport on any level of nested subsystems to allow NI VeriStand software to map signals to it.
      mask init:
      | NIVeriStandIO_init;
      settings: CopyFcn=NIVeriStand_MDL_functions('', 'IO_copy');  DeleteFcn=NIVeriStand_MDL_functions('', 'IO_delete');  MoveFcn=set_param(gcb, 'Mask', 'on');
      mask Callback portnum: NIVeriStand_MDL_functions('', 'IO_setportnum');
      mask TypeOptions dtype: auto | double | single | int8 | uint8 | int16 | uint16 | int32 | uint32 | boolean
      mask Callback dtype: NIVeriStand_MDL_functions('', 'IO_booleansignal');
      mask TypeOptions stype: auto | real | complex
      mask Display:
      | patch([-x x], [-y y], [.90980 .81960 .32156]);
      | plot([xrad -x x xrad], [yrad -y y yrad]);
      | fprintf('NI Out%d', portnum);
  y_tilde : S-Function  Priority=2  FunctionName=NIVeriStandIO  Parameters=width dtype portnum stime stype btype  SFunctionDeploymentMode=off  EnableBusSupport=off  mask(NI VeriStand Outport){portnum=2, width=-1, stime=-1, dtype=auto, stype=auto, btype=0}
      mask prompts: portnum "Port number:"; width "Port dimensions (-1 for dynamically sized):"; stime "Sample time (-1 for inherited):"; dtype "Data type:"; stype "Signal type:"; btype "Block type:"
      mask help: Use this outport on any level of nested subsystems to allow NI VeriStand software to map signals to it.
      mask init:
      | NIVeriStandIO_init;
      settings: CopyFcn=NIVeriStand_MDL_functions('', 'IO_copy');  DeleteFcn=NIVeriStand_MDL_functions('', 'IO_delete');  MoveFcn=set_param(gcb, 'Mask', 'on');
      mask Callback portnum: NIVeriStand_MDL_functions('', 'IO_setportnum');
      mask TypeOptions dtype: auto | double | single | int8 | uint8 | int16 | uint16 | int32 | uint32 | boolean
      mask Callback dtype: NIVeriStand_MDL_functions('', 'IO_booleansignal');
      mask TypeOptions stype: auto | real | complex
      mask Display:
      | patch([-x x], [-y y], [.90980 .81960 .32156]);
      | plot([xrad -x x xrad], [yrad -y y yrad]);
      | fprintf('NI Out%d', portnum);
  wires:
  eta_tilde/1 -> Demux/1
  Demux/2 -> y_tilde/1
  Demux/3 -> psi_tilde/1
  Demux/1 -> x_tilde/1

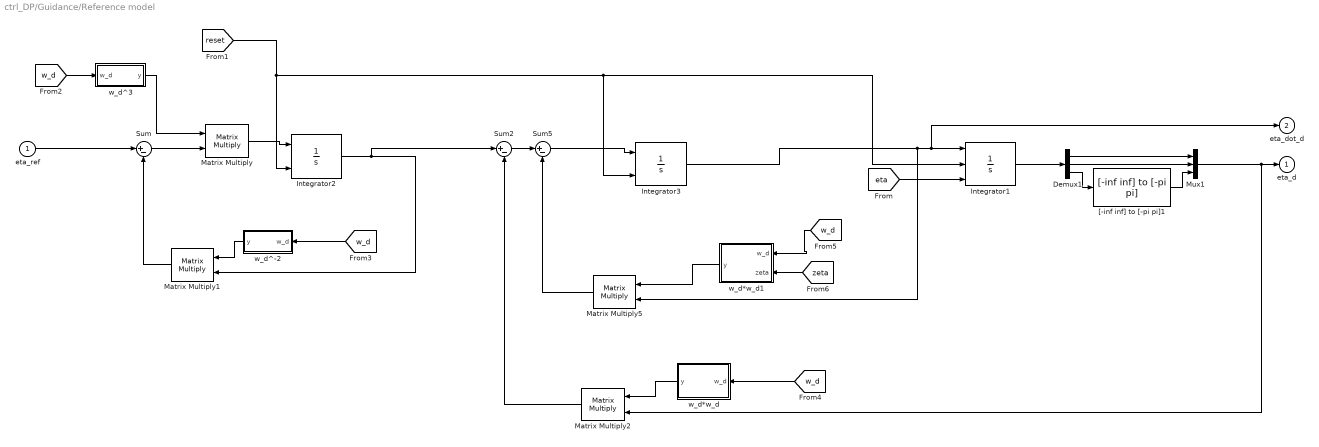
== system ctrl_DP/Guidance/Reference model ==
  eta_ref : Inport
  Demux1 : Demux  Outputs=3
  Integrator1 : Integrator  ExternalReset=either  InitialConditionSource=external
  Integrator2 : Integrator  ExternalReset=either
  Integrator3 : Integrator  ExternalReset=either
  Matrix Multiply{,1..2,5} (4 alike) : Product  Multiplication=Matrix(*)
  Mux1 : Mux  Inputs=3
  Sum : Sum  Inputs=|+-
  Sum2 : Sum  Inputs=|+-  SaturateOnIntegerOverflow=on  InputSameDT=on  OutDataTypeStr=Inherit: Same as first input
  Sum5 : Sum  Inputs=|+-  SaturateOnIntegerOverflow=on  InputSameDT=on  OutDataTypeStr=Inherit: Same as first input
  "[-inf inf] to [-pi pi]1" : marine_gnc/Utilities/Math Operations/[-inf inf] to [-pi pi]
  w_d*w_d : MATLAB Function  TreatAsAtomicUnit=on
  w_d*w_d1 : MATLAB Function  TreatAsAtomicUnit=on
  w_d^-2 : MATLAB Function  TreatAsAtomicUnit=on
  w_d^3 : MATLAB Function  TreatAsAtomicUnit=on
  eta_d : Outport  InitialOutput=0
  eta_dot_d : Outport  Port=2  InitialOutput=0
  wires:
  Integrator3/1 -> eta_dot_d/1, Integrator1/1, Matrix Multiply5/2
  Sum5/1 -> Integrator3/1
  Integrator2/1 -> Sum2/1, Matrix Multiply1/2
  Sum2/1 -> Sum5/1
  Matrix Multiply2/1 -> Sum2/2
  Mux1/1 -> Matrix Multiply2/2, eta_d/1
  Matrix Multiply5/1 -> Sum5/2
  eta_ref/1 -> Sum/1
  Sum/1 -> Matrix Multiply/2
  Matrix Multiply/1 -> Integrator2/1
  Matrix Multiply1/1 -> Sum/2
  [w_d] -> w_d^3/1(w_d)
  [w_d] -> w_d^-2/1(w_d)
  [w_d] -> w_d*w_d/1(w_d)
  w_d*w_d/1(y) -> Matrix Multiply2/1
  [zeta] -> w_d*w_d1/2(zeta)
  [w_d] -> w_d*w_d1/1(w_d)
  w_d*w_d1/1(y) -> Matrix Multiply5/1
  [eta] -> Integrator1/3
  [reset] -> Integrator3/2, Integrator1/2, Integrator2/2
  w_d^-2/1(y) -> Matrix Multiply1/1
  w_d^3/1(y) -> Matrix Multiply/1
  Demux1/1 -> Mux1/1
  "[-inf inf] to [-pi pi]1"/1 -> Mux1/3
  Demux1/3 -> "[-inf inf] to [-pi pi]1"/1
  Demux1/2 -> Mux1/2
  Integrator1/1 -> Demux1/1

== system ctrl_DP/Nonlinear Passisve Observer/Transpose Rotation Matrix ==
  psi : Inport
  y_tilde : Inport  Port=2
  Mux : Mux  Inputs=2
  Mux1 : Mux  Inputs=3
  Row1 : Fcn  Expr=cos(u(1))*u(2)+sin(u(1))*u(3)
  Row2 : Fcn  Expr=-sin(u(1))*u(2)+cos(u(1))*u(3)
  Row3 : Fcn  Expr=u(4)
  R(psi)'*y_tilde : Outport
  wires:
  Mux/1 -> Row3/1, Row2/1, Row1/1
  Row1/1 -> Mux1/1
  Row2/1 -> Mux1/2
  Row3/1 -> Mux1/3
  Mux1/1 -> R(psi)'*y_tilde/1
  psi/1 -> Mux/1
  y_tilde/1 -> Mux/2

== system ctrl_DP/Nonlinear Passisve Observer/Transpose Rotation matrix ==
  psi : Inport
  b_hat : Inport  Port=2
  Mux : Mux  Inputs=2
  Mux1 : Mux  Inputs=3
  Row1 : Fcn  Expr=cos(u(1))*u(2)+sin(u(1))*u(3)
  Row2 : Fcn  Expr=-sin(u(1))*u(2)+cos(u(1))*u(3)
  Row3 : Fcn  Expr=u(4)
  R(psi)'*b_hat : Outport
  wires:
  Mux/1 -> Row3/1, Row2/1, Row1/1
  Row1/1 -> Mux1/1
  Row2/1 -> Mux1/2
  Row3/1 -> Mux1/3
  Mux1/1 -> R(psi)'*b_hat/1
  psi/1 -> Mux/1
  b_hat/1 -> Mux/2
